simulink model "Part4_1_eqn1"  (R2021a)
settings: Solver=VariableStepAuto  StartTime=0.0  StopTime=100  RelTol=1e-3
settings Model: Creator=theod  LastModifiedBy=theod

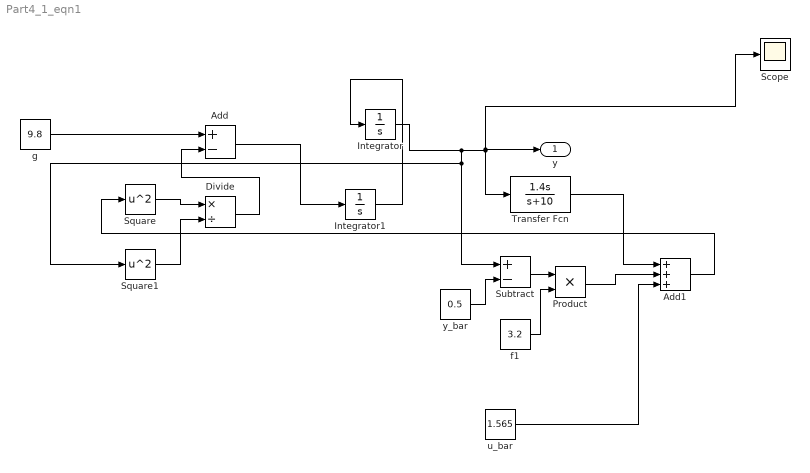
== system Part4_1_eqn1 ==
  Add : Sum  Inputs=+-
  Add1 : Sum  Inputs=+++
  Divide : Product  Inputs=*/
  Integrator : Integrator  InitialCondition=1.3
  Integrator1 : Integrator  InitialCondition=0.5
  Product : Product
  Scope : Scope
  Square : Math  Operator=square  SaturateOnIntegerOverflow=on
  Square1 : Math  Operator=square  SaturateOnIntegerOverflow=on
  Subtract : Sum  Inputs=+-
  Transfer Fcn : TransferFcn  Numerator=[1.4 0]  Denominator=[1 10]
  f1 : Constant  Value=3.2
  g : Constant  Value=9.8
  u_bar : Constant  Value=1.565
  y_bar : Constant  Value=0.5
  y : Outport
  wires:
  Integrator1/1 -> Integrator/1
  Square/1 -> Divide/1
  Square1/1 -> Divide/2
  Divide/1 -> Add/2
  g/1 -> Add/1
  Add/1 -> Integrator1/1
  f1/1 -> Product/2
  Product/1 -> Add1/2
  u_bar/1 -> Add1/3
  Add1/1 -> Square/1
  y_bar/1 -> Subtract/2
  Integrator/1 -> Square1/1, Subtract/1, Scope/1, y/1, Transfer Fcn/1
  Subtract/1 -> Product/1
  Transfer Fcn/1 -> Add1/1
